simulink model "QArm_Lab2"  (R2022a)
settings: Solver=ode4  StartTime=0.0  StopTime=inf  FixedStep=1/500  RelTol=1e-3  EnableMultiTasking=on
undefined symbols (not defined in the file): HIL, qc_get_step_size
libraries: quarc_library x8, simulink_extras x2, simulink x1
settings Model: SimulationMode=external  ExtModeTrigDuration=10000  Creator=fvranes  LastModifiedBy=niraj
settings SolverCC: AlgebraicLoopSolver=TrustRegion  PositivePriorityOrder=on
settings DataIOCC: SaveOutput=off  SignalLogging=off  DSMLogging=off  SaveTime=off  ReturnWorkspaceOutputs=off
settings OptimizationCC: LifeSpan=inf
settings DebuggingCC: UnconnectedInputMsg=warning  UnconnectedOutputMsg=warning  UnconnectedLineMsg=warning  SFMachineParentedDataDiag=warning  ArithmeticOperatorsInVariantConditions=warning
settings SFSimCC: SimUseLocalCustomCode=off  CustomCodeUndefinedFunction=UseInterfaceOnly
settings RTWCC: Description=QUARC Win64 Target  SystemTargetFile=quarc_win64.tlc  TemplateMakefile=quarc_default_tmf  RTWUseLocalCustomCode=off  DLArmComputeVersion=19.05
settings CodeAppCC: StateflowObjectComments=on
settings STFCustomTargetCC: TargetPreCompLibLocation=C:\PROGRA~3\QUARC\lib\2021a\win64\debug  TargetLangStandard=C99 (ISO)  ConcurrentExecutionCompliant=on  SystemTargetFile=quarc_win64.tlc
settings GRTTargetCC: TargetPreCompLibLocation=C:\PROGRA~3\QUARC\lib\2021a\win64\debug  ParMdlRefBuildCompliant=off  CompOptLevelCompliant=off  CombineOutputUpdateFcns=off  MatFileLogging=off  CPPClassGenCompliant=off  GRTInterface=on  UseToolchainInfoCompliant=off  ExtMode=on  ExtModeMexFile=quarc_comm
settings ConfigComp: CovMetricSettings=dswe

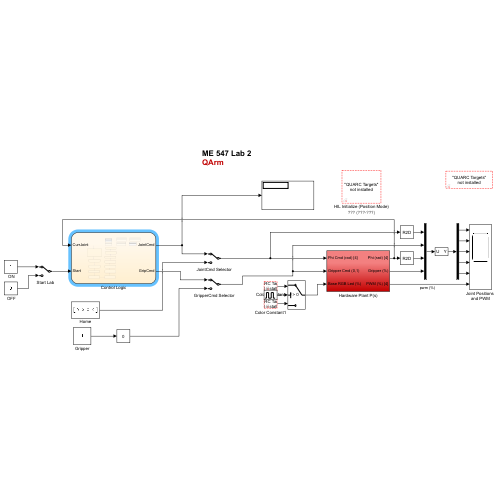
[thumbnail: Simulink's stored preview of the top-level diagram]
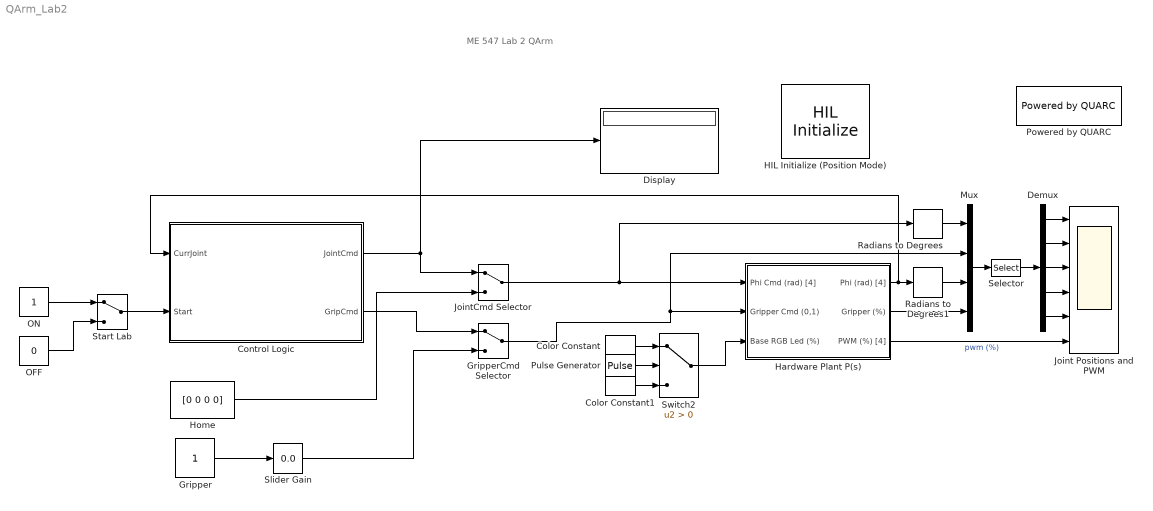
== system QArm_Lab2 ==
  note: ME 547 Lab 2
      | QArm
  " OFF" : Constant  Value=0
  " ON" : Constant
  Color Constant : quarc_library/Sources/Signals/Color Constant  color=[0 1 0]
      settings: SourceProductName=QUARC Targets
  Color Constant1 : quarc_library/Sources/Signals/Color Constant  color=[0 0 1]
      settings: SourceProductName=QUARC Targets
  Control Logic : Stateflow chart  TreatAsAtomicUnit=on
  Demux : Demux  Outputs=[2 2 2 2 2]
  Display : Display
  Gripper : Constant
  GripperCmd Selector : ManualSwitch
  HIL Initialize (Position Mode) : quarc_library/Data Acquisition/Generic/Configuration/HIL Initialize  object_name=HIL-1  board_type=qarm_usb  board_number=0  board_options=j0_mode=0;j1_mode=0;j2_mode=0;j3_mode=0;gripper_mode=0;j0_profile_config=0;j0_profile_velocity=1.5708;j0_profile_acceleration=1.0472;j1_profile_config=0;j1_profile_velocity=1.5708;j1_profile_acceleration=1.0472;j2_profile_config=0;j2_profile_velocity=1.5708;j2_profile_acceleration=1.0472;j3_profile_config=0;j3_profile_velocity=1.5708;j3_profile_acceleration=1.0472;  exclusive=off  active=on  hardware_clocks=[0]  clock_modes=[]  initial_clock_frequencies=[]  set_clock_params_at_start=off  set_clock_params_at_switch_in=off  set_clock_frequencies_at_start=off  set_clock_frequencies_at_switch_in=off  analog_input_channels=[5:9]  analog_input_configurations=[]  analog_input_maximums=[]  analog_input_minimums=[]  set_analog_input_params_at_start=off  set_analog_input_params_at_switch_in=off  analog_output_channels=[]  analog_output_maximums=[]  analog_output_minimums=[]  initial_analog_outputs=[]  final_analog_outputs=[]  watchdog_analog_outputs=[]  set_analog_output_params_at_start=off  set_analog_output_params_at_switch_in=off  set_analog_outputs_at_start=off  set_analog_outputs_at_switch_in=off  set_analog_outputs_at_terminate=off  set_analog_outputs_at_switch_out=off  set_analog_outputs_on_watchdog=off  digital_input_channels=[]  digital_output_channels=[]  digital_output_configuration=[]  initial_digital_outputs=[]  final_digital_outputs=[]  watchdog_digital_outputs=[]  set_digital_output_params_at_start=off  set_digital_output_params_at_switch_in=off  set_digital_outputs_at_start=off  set_digital_outputs_at_switch_in=off  set_digital_outputs_at_terminate=off  set_digital_outputs_at_switch_out=off  set_digital_outputs_on_watchdog=off  encoder_channels=[]  quadrature=[]  encoder_filter_frequency=[]  initial_encoder_counts=[]  set_encoder_params_at_start=off  set_encoder_params_at_switch_in=off  set_encoder_counts_at_start=off  set_encoder_counts_at_switch_in=off  pwm_channels=[]  pwm_modes=[]  pwm_frequency=[]  pwm_configuration=[]  pwm_alignment=[]  pwm_polarity=[]  pwm_leading_deadband=[]  pwm_trailing_deadband=[]  initial_pwm_outputs=[]  final_pwm_outputs=[]  watchdog_pwm_outputs=[]  set_pwm_params_at_start=off  set_pwm_params_at_switch_in=off  set_pwm_outputs_at_start=off  set_pwm_outputs_at_switch_in=off  set_pwm_outputs_at_terminate=off  set_pwm_outputs_at_switch_out=off  set_pwm_outputs_on_watchdog=off  other_output_channels=[1000:1004 11000:11008]  initial_other_outputs=[0]  final_other_outputs=[0]  watchdog_other_outputs=[]  set_other_outputs_at_start=on  set_other_outputs_at_switch_in=off  set_other_outputs_at_terminate=on  set_other_outputs_at_switch_out=off  set_other_outputs_on_watchdog=off
  Hardware Plant P(s) : Subsystem
  Home : Constant  Value=[0 0 0 0]
  Joint Positions and PWM : Scope  NumInputPorts=6
  JointCmd Selector : ManualSwitch
  Mux : Mux
  Powered by QUARC : quarc_library/Logos/Powered by QUARC
  Pulse Generator : DiscretePulseGenerator  PulseType=Time based  Period=1  PulseWidth=50
  Radians to Degrees : simulink_extras/Transformations/Radians to Degrees
  Radians to Degrees1 : simulink_extras/Transformations/Radians to Degrees
  Selector : Selector  InputPortWidth=10  IndexOptions=Index vector (dialog)  Indices=[1 6 2 7 3 8 4 9 5 10]  OutputSizes=1
  Slider Gain : simulink/Math Operations/Slider Gain  gain=0.0  low=0  high=1
  Start Lab : ManualSwitch
  Switch2 : Switch  Criteria=u2 > Threshold  SaturateOnIntegerOverflow=off  InputSameDT=off
  wires:
  Switch2/1 -> Hardware Plant P(s)/3(Base RGB Led (%))
  Hardware Plant P(s)/2(Gripper (%)) -> Mux/4
  Mux/1 -> Selector/1
  Hardware Plant P(s)/3(PWM (%) [4]) -> Joint Positions and PWM/6  "pwm (%)"
  Radians to Degrees/1 -> Mux/1
  Radians to Degrees1/1 -> Mux/3
  Selector/1 -> Demux/1
  Demux/1 -> Joint Positions and PWM/1
  Demux/2 -> Joint Positions and PWM/2
  Demux/3 -> Joint Positions and PWM/3
  Demux/4 -> Joint Positions and PWM/4
  Demux/5 -> Joint Positions and PWM/5
  Color Constant/1 -> Switch2/1
  Color Constant1/1 -> Switch2/3
  Pulse Generator/1 -> Switch2/2
  Start Lab/1 -> Control Logic/2(Start)
  Control Logic/1(JointCmd) -> Display/1, JointCmd Selector/1
  Control Logic/2(GripCmd) -> GripperCmd Selector/1
  JointCmd Selector/1 -> Radians to Degrees/1, Hardware Plant P(s)/1(Phi Cmd (rad) [4])
  GripperCmd Selector/1 -> Mux/2, Hardware Plant P(s)/2(Gripper Cmd (0,1))
  Home/1 -> JointCmd Selector/2
  Slider Gain/1 -> GripperCmd Selector/2
  " OFF"/1 -> Start Lab/2
  " ON"/1 -> Start Lab/1
  Hardware Plant P(s)/1(Phi (rad) [4]) -> Control Logic/1(CurrJoint), Radians to Degrees1/1
  Gripper/1 -> Slider Gain/1

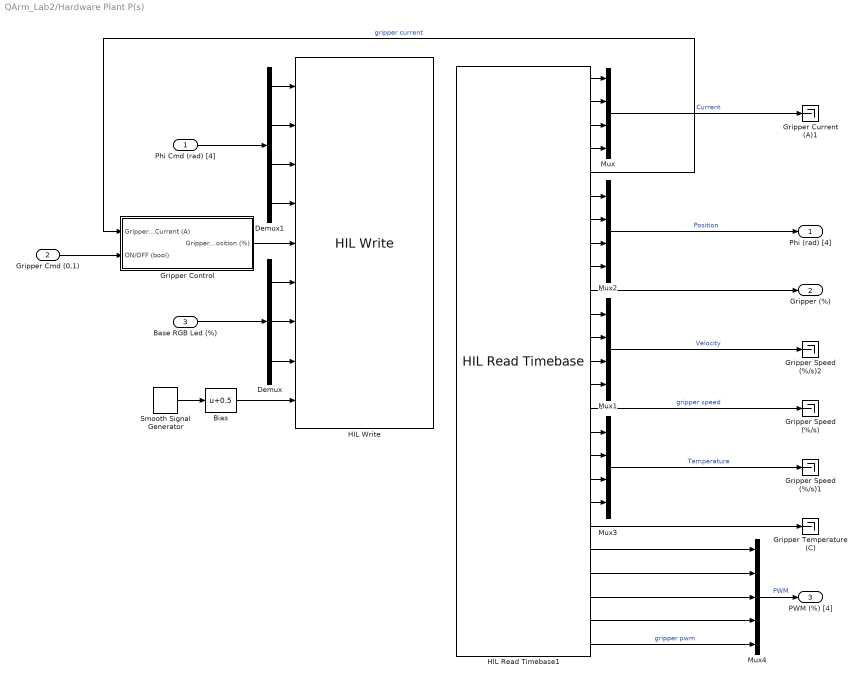
== system QArm_Lab2/Hardware Plant P(s) ==
  Phi Cmd (rad) [4] : Inport
  Gripper Cmd (0,1) : Inport  Port=2
  Base RGB Led (%) : Inport  Port=3
  Bias : Bias  Bias=0.5  SaturateOnIntegerOverflow=off
  Demux : Demux  Outputs=3
  Demux1 : Demux
  Gripper Control : Subsystem
  Gripper Current (A)1 : Terminator
  Gripper Speed (%/s) : Terminator
  Gripper Speed (%/s)1 : Terminator
  Gripper Speed (%/s)2 : Terminator
  Gripper Temperature (C) : Terminator
  HIL Read Timebase1 : quarc_library/Data Acquisition/Generic/Timebases/HIL Read Timebase  object_name=HIL-1  clock=0  analog_channels=[5:9]  encoder_channels=[]  digital_channels=[]  other_channels=[1000:1004 3000:3004 10000:10004 11000:11004]  active=on  vector_output=off  data_type_mode=Inherit via back propagation  encoder_data_type=double  digital_data_type=boolean  overflow_mode=Error on overflow  samples_in_buffer=max(ceil(1/qc_get_step_size), 1)
  HIL Write : quarc_library/Data Acquisition/Generic/Immediate I//O/HIL Write  object_name=HIL-1  analog_channels=[]  pwm_channels=[]  digital_channels=[]  other_channels=[1000:1004 11005:11008]  sample_time=-1  active=on  vector_input=off
  Mux{,1..3} (4 alike) : Mux
  Mux4 : Mux  Inputs=5
  Smooth Signal Generator : quarc_library/Sources/Signals/Smooth Signal Generator  signal_type=Sine  source=Internal (dialog parameters)  amplitude=0.5  frequency=60/72  initial_phase=0  sample_time=qc_get_step_size  output_cos=off
      settings: SourceProductName=QUARC Targets
  Phi (rad) [4] : Outport  VectorParamsAs1DForOutWhenUnconnected=off
  Gripper (%) : Outport  Port=2  VectorParamsAs1DForOutWhenUnconnected=off
  PWM (%) [4] : Outport  Port=3  VectorParamsAs1DForOutWhenUnconnected=off
  wires:
  HIL Read Timebase1/10 -> Gripper (%)/1
  Mux4/1 -> PWM (%) [4]/1  "PWM"
  HIL Read Timebase1/25 -> Mux4/5  "gripper pwm"
  HIL Read Timebase1/24 -> Mux4/4
  HIL Read Timebase1/23 -> Mux4/3
  HIL Read Timebase1/22 -> Mux4/2
  HIL Read Timebase1/21 -> Mux4/1
  Mux2/1 -> Phi (rad) [4]/1  "Position"
  Phi Cmd (rad) [4]/1 -> Demux1/1
  Demux1/4 -> HIL Write/4
  Demux1/3 -> HIL Write/3
  Demux1/2 -> HIL Write/2
  Demux1/1 -> HIL Write/1
  Base RGB Led (%)/1 -> Demux/1
  Mux3/1 -> Gripper Speed (%/s)1/1  "Temperature"
  Mux1/1 -> Gripper Speed (%/s)2/1  "Velocity"
  Mux/1 -> Gripper Current (A)1/1  "Current"
  HIL Read Timebase1/20 -> Gripper Temperature (C)/1
  HIL Read Timebase1/1 -> Mux/1
  HIL Read Timebase1/2 -> Mux/2
  HIL Read Timebase1/13 -> Mux1/3
  Demux/2 -> HIL Write/7
  HIL Read Timebase1/19 -> Mux3/4
  Demux/1 -> HIL Write/6
  HIL Read Timebase1/11 -> Mux1/1
  HIL Read Timebase1/16 -> Mux3/1
  HIL Read Timebase1/17 -> Mux3/2
  HIL Read Timebase1/3 -> Mux/3
  Demux/3 -> HIL Write/8
  HIL Read Timebase1/15 -> Gripper Speed (%/s)/1  "gripper speed"
  HIL Read Timebase1/5 -> Gripper Control/1(Gripper Current (A))  "gripper current"
  HIL Read Timebase1/7 -> Mux2/2
  HIL Read Timebase1/4 -> Mux/4
  HIL Read Timebase1/12 -> Mux1/2
  HIL Read Timebase1/8 -> Mux2/3
  HIL Read Timebase1/18 -> Mux3/3
  HIL Read Timebase1/6 -> Mux2/1
  HIL Read Timebase1/9 -> Mux2/4
  HIL Read Timebase1/14 -> Mux1/4
  Gripper Control/1(Gripper Position (%)) -> HIL Write/5
  Gripper Cmd (0,1)/1 -> Gripper Control/2(ON/OFF (bool))
  Smooth Signal Generator/1 -> Bias/1
  Bias/1 -> HIL Write/9

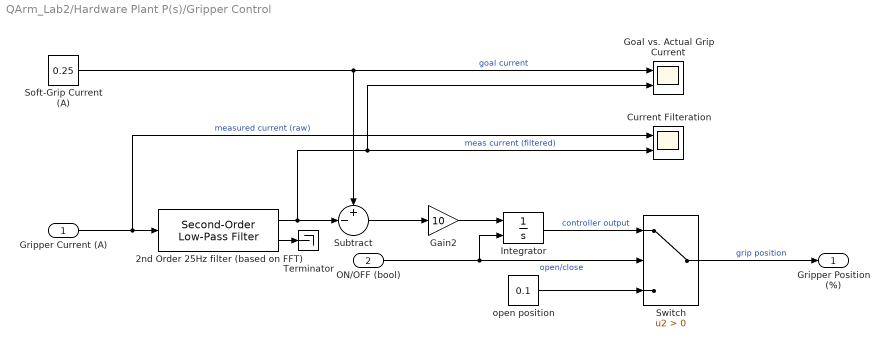
== system QArm_Lab2/Hardware Plant P(s)/Gripper Control ==
  Gripper Current (A) : Inport
  ON/OFF (bool) : Inport  Port=2
  2nd Order 25Hz filter (based on FFT) : quarc_library/Continuous/Second-Order Low-Pass Filter  params_source=Internal (dialog parameters)  input_width=25*2*pi  input_zeta=1  input_init=0
  Current Filteration : Scope  NumInputPorts=2
  Gain2 : Gain  Gain=10
  Goal vs. Actual Grip Current : Scope  NumInputPorts=2
  Integrator : Integrator  ExternalReset=either  InitialCondition=0.1  LimitOutput=on  UpperSaturationLimit=0.9  LowerSaturationLimit=0.1
  Soft-Grip Current (A) : Constant  Value=0.25
  Subtract : Sum  Inputs=+-|
  Switch : Switch  Criteria=u2 > Threshold  SaturateOnIntegerOverflow=off  InputSameDT=off
  Terminator : Terminator
  open position : Constant  Value=0.1
  Gripper Position (%) : Outport  VectorParamsAs1DForOutWhenUnconnected=off
  wires:
  Gripper Current (A)/1 -> 2nd Order 25Hz filter (based on FFT)/1, Current Filteration/1  "measured current (raw)"
  ON/OFF (bool)/1 -> Switch/2, Integrator/2  "open/close"
  open position/1 -> Switch/3
  Switch/1 -> Gripper Position (%)/1  "grip position"
  Soft-Grip Current (A)/1 -> Subtract/1, Goal vs. Actual Grip Current/1  "goal current"
  2nd Order 25Hz filter (based on FFT)/1 -> Subtract/2, Current Filteration/2, Goal vs. Actual Grip Current/2  "meas current (filtered)"
  Subtract/1 -> Gain2/1
  Integrator/1 -> Switch/1  "controller output"
  Gain2/1 -> Integrator/1
  2nd Order 25Hz filter (based on FFT)/2 -> Terminator/1

== stateflow chart QArm_Lab2/Control Logic ==
  state Home
    entry:
    JointCmd = [0, 0, 0, 0];
  state Start
    entry:
    % DH parameters
    a = [0, sqrt(350^2+50^2), 0, 0];
    alpha = [-pi/2, 0, -pi/2, 0];
    d = [140, 0, 0, 360];
    % Joint angles in rad
    A = []; %xyz = 400, 400, 150
    B = []; %xyz = 400, 400, 110
    C = []; %xyz = 450, 200, 300
    D = []; %xyz = 500, 0, 350
    E = []; %xyz = 600, -100, 200
    F = []; %xyz = 600, -100, 135
  state MoveBackToE
    entry:
    JointCmd = DH2Sim(E);
  state OpenGripper
    entry:
    GripCmd = 0;
  state MoveToA
    entry:
    JointCmd = DH2Sim(A);
  state MoveToF
    entry:
    JointCmd = DH2Sim(F);
  state MoveToB
    entry:
    JointCmd = DH2Sim(B);
  state MoveToE
    entry:
    JointCmd = DH2Sim(E);
  state MoveToD
    entry:
    JointCmd = DH2Sim(D);
  state CloseGripper
    entry:
    GripCmd = 0.8;
  state MoveBackToA
    entry:
    JointCmd = DH2Sim(A);
  state MoveToC
    entry:
    JointCmd = DH2Sim(C);
  (default) -> Start
  MoveBackToE -> Home : [after(5, sec)]
  OpenGripper -> MoveBackToE : [after(5, sec)]
  Start -> MoveToA : [after(5, sec)&&Start==1]
  MoveToF -> OpenGripper : [after(5, sec)]
  MoveToA -> MoveToB : [after(5, sec)]
  MoveToE -> MoveToF : [after(5, sec)]
  MoveToB -> CloseGripper : [after(5, sec)]
  MoveToD -> MoveToE : [after(3, sec)]
  CloseGripper -> MoveBackToA : [after(5, sec)]
  MoveToC -> MoveToD : [after(3, sec)]
  MoveBackToA -> MoveToC : [after(5, sec)]
  data: index function_input; TransMatrix function_output; theta function_input; flag function_output; threshold function_input; actual function_input; target function_input; DHAng function_input; SimAng function_output; T1 function_input; CurrPosition function_output; T2 function_input; T3 function_input; T4 function_input; SimAng function_input; DHAng function_output; Pos function_input; JTarget function_output; CurrJoint input; JointCmd output; a local; alpha local; d local; JointTarget local; Start input; GripCmd output; A local; B local; C local; D local; E local; F local
  function TransMatrix = FrameTrans(index, theta):
    | function TransMatrix = FrameTrans(index, theta)
    | TransMatrix = [cos(theta(index)), -sin(theta(index))*cos(alpha(index)), sin(theta(index))*sin(alpha(index)), a(index)*cos(theta(index)); ... 
    |                sin(theta(index)), cos(theta(index))*cos(alpha(index)), -cos(theta(index))*sin(alpha(index)), a(index)*sin(theta(index)); ...
    |                0, sin(alpha(index)), cos(alpha(index)), d(index); ...
    |                0, 0, 0, 1];
    | end
  function flag = checkThres(threshold, actual, target):
    | function flag = checkThres(threshold, actual, target)
    | diff = abs(actual-target);
    | max_diff = max(diff, [], 'all');
    | if max_diff <= threshold
    |     flag = 1;
    | else
    |     flag = 0;
    | end
    | end
  function SimAng = DH2Sim(DHAng):
    | function SimAng = DH2Sim(DHAng)
    | SimAng = [0, 0, 0, 0];
    | SimAng(1) = DHAng(1);
    | SimAng(2) = DHAng(2)+atan(0.35/0.05);
    | SimAng(3) = DHAng(3)+atan(0.05/0.35);
    | SimAng(4) = DHAng(4);
    | end
  function CurrPosition = FKine(T1, T2, T3, T4):
    | function CurrPosition = FKine(T1, T2, T3, T4)
    | T04 = T1*T2*T3*T4;
    | CurrPosition = [T04(1, 4), T04(2, 4), T04(3, 4)];
    | end
  function DHAng = Sim2DH(SimAng):
    | function DHAng = Sim2DH(SimAng)
    | DHAng = [0, 0, 0, 0];
    | DHAng(1) = SimAng(1);
    | DHAng(2) = SimAng(2)-atan(0.35/0.05);
    | DHAng(3) = SimAng(3)-atan(0.05/0.35);
    | DHAng(4) = SimAng(4);
    | end
  function JTarget = IKine(Pos):
    | function JTarget = IKine(Pos)
    | xc = Pos(1);
    | yc = Pos(2);
    | zc = Pos(3);
    | 
    | theta1 = atan2(yc, xc);
    | 
    | r = sqrt(xc^2+yc^2);
    | s = zc-d(1);
    | D = sqrt(r^2+s^2);
    | F = (D^2-a(2)^2-d(4)^2)/(2*a(2)*d(4));
    | ang = atan2(sqrt((1-F^2)), F); % force elbow up
    | theta3 = -(pi/2-ang);
    | 
    | delta = atan2(d(4)*sin(ang), a(2)+d(4)*cos(ang));
    | theta2 = -(atan2(s,r)+delta);
    | 
    | JTarget = [theta1, theta2, theta3, 0];
    | end
